simulink model "model"  (R2024b)
settings: Solver=VariableStepAuto  StartTime=0.0  StopTime=inf  RelTol=1e-3
StopFcn:
  | try
  |     delete(instrfindall);
  |     fclose(instrfindall);
  | catch
  | end
libraries: simulink x4, instrumentseriallib x3
settings Model: Creator=andre  LastModifiedBy=andre

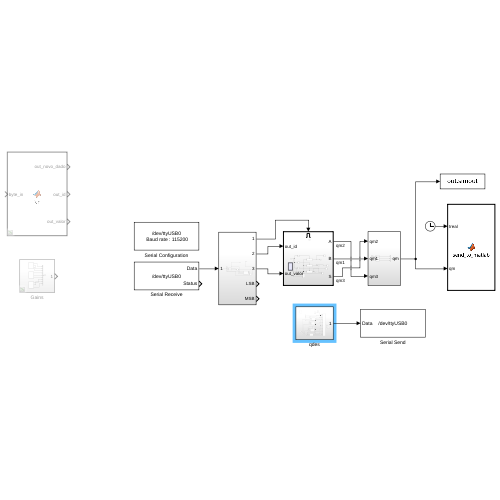
[thumbnail: Simulink's stored preview of the top-level diagram]
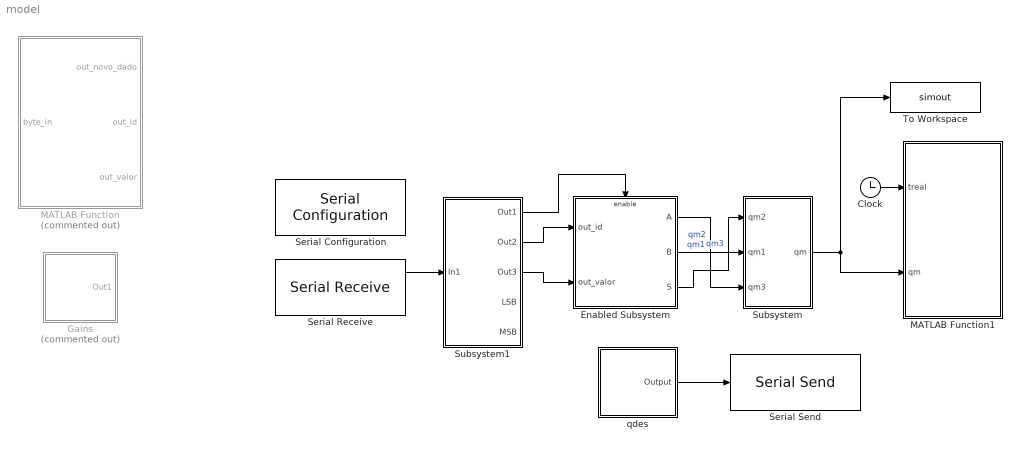
== system model ==
  Clock : Clock
  Enabled Subsystem : Subsystem  TreatAsAtomicUnit=on
  Gains : Subsystem  Commented=on
  MATLAB Function : MATLAB Function  Commented=on  TreatAsAtomicUnit=on
  MATLAB Function1 : MATLAB Function  TreatAsAtomicUnit=on
  Serial Configuration : instrumentseriallib/Serial Configuration  Priority=-200000  PortSel=/dev/ttyUSB0  Port=/dev/ttyUSB0  ComPort=/dev/ttyUSB0  BaudRate=115200  DataBits=8  Parity=none  StopBits=1  ByteOrder=little-endian  FlowControl=none  Timeout=10  SimulateUsing=Interpreted execution  BlockInModel=on  aMode=1
  Serial Receive : instrumentseriallib/Serial Receive  Priority=1  PortSel=/dev/ttyUSB0  Port=/dev/ttyUSB0  ComPort=/dev/ttyUSB0  DataType=uint8  SaveDataType=uint8  ToggleHeader=on  Header=[170]  ToggleDataSize=on  DataSize=[5 1]  ToggleTerminator=on  Terminator=Custom terminator  CustomTerminator=[187]  InputFormat=Column major  EnableBlockingMode=off  ActionDataUnavailable=Output last received value  ActionWhenDataUnavailable=Output last received value  CustomValue=0  SampleTime=0.001  SimulateUsing=Interpreted execution  BlockInModel=on  aMode=1
  Serial Send : instrumentseriallib/Serial Send  Priority=1  PortSel=/dev/ttyUSB0  Port=/dev/ttyUSB0  ComPort=/dev/ttyUSB0  Header=[]  Terminator=<none>  CustomTerminator=[]  EnableBlockingMode=off  SimulateUsing=Interpreted execution  BlockInModel=on  aMode=1
  Subsystem : Subsystem
  Subsystem1 : Subsystem
  To Workspace : ToWorkspace  VariableName=simout  SaveFormat=Timeseries  SampleTime=-1
  qdes : Subsystem
  wires:
  Clock/1 -> MATLAB Function1/1(treal)
  Enabled Subsystem/2(B) -> Subsystem/2(qm1)  "qm1"
  Subsystem/1(qm) -> To Workspace/1, MATLAB Function1/2(qm)
  qdes/1(Output) -> Serial Send/1
  Enabled Subsystem/3(S) -> Subsystem/1(qm2)  "qm3"
  Enabled Subsystem/1(A) -> Subsystem/3(qm3)  "qm2"
  Serial Receive/1 -> Subsystem1/1(In1)
  Subsystem1/1(Out1) -> Enabled Subsystem/Enable
  Subsystem1/2(Out2) -> Enabled Subsystem/1(out_id)
  Subsystem1/3(Out3) -> Enabled Subsystem/2(out_valor)

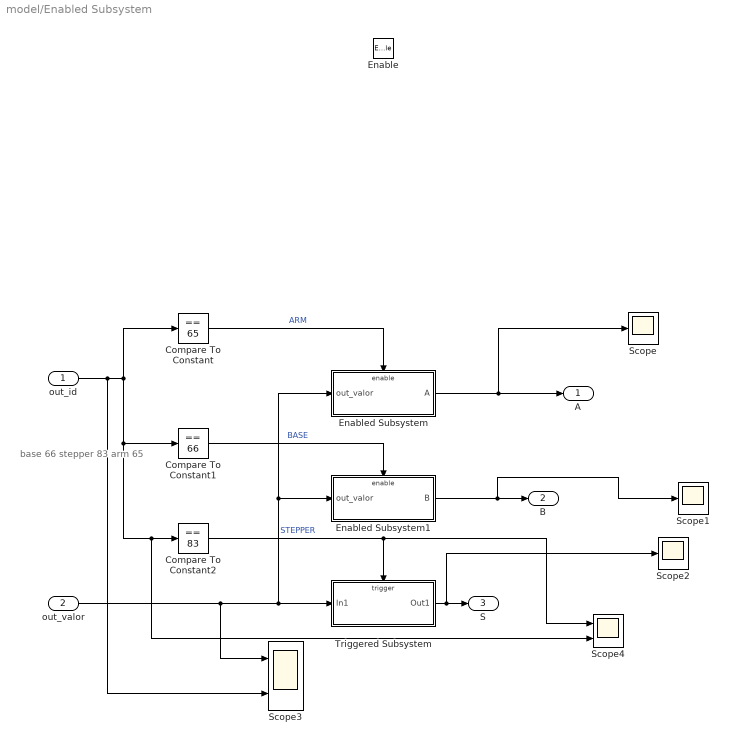
== system model/Enabled Subsystem ==
  note: base 66
      | stepper 83
      | arm 65
  out_id : Inport
  out_valor : Inport  Port=2
  Enable : EnablePort
  Compare To Constant : simulink/Logic and Bit Operations/Compare To Constant  relop===  const=65  OutDataTypeStr=boolean
  Compare To Constant1 : simulink/Logic and Bit Operations/Compare To Constant  relop===  const=66  OutDataTypeStr=boolean
  Compare To Constant2 : simulink/Logic and Bit Operations/Compare To Constant  relop===  const=83  OutDataTypeStr=boolean
  Enabled Subsystem : Subsystem  TreatAsAtomicUnit=on
  Enabled Subsystem1 : Subsystem  TreatAsAtomicUnit=on
  Scope : Scope
  Scope1 : Scope
  Scope2 : Scope
  Scope3 : Scope  NumInputPorts=2
  Scope4 : Scope  NumInputPorts=2
  Triggered Subsystem : Subsystem  TreatAsAtomicUnit=on
  A : Outport
  B : Outport  Port=2
  S : Outport  Port=3
  wires:
  Compare To Constant/1 -> Enabled Subsystem/Enable  "ARM"
  Triggered Subsystem/1(Out1) -> Scope2/1, S/1
  Compare To Constant2/1 -> Scope4/1, Triggered Subsystem/Trigger  "STEPPER"
  out_id/1 -> Scope3/2, Scope4/2, Compare To Constant2/1, Compare To Constant1/1, Compare To Constant/1
  out_valor/1 -> Scope3/1, Triggered Subsystem/1(In1), Enabled Subsystem/1(out_valor), Enabled Subsystem1/1(out_valor)
  Compare To Constant1/1 -> Enabled Subsystem1/Enable  "BASE"
  Enabled Subsystem/1(A) -> Scope/1, A/1
  Enabled Subsystem1/1(B) -> Scope1/1, B/1

== system model/Gains ==
  D_gain : Subsystem
  I_gain : Subsystem
  P_gain : Subsystem
  Vector Concatenate : Concatenate  NumInputs=9
  Out1 : Outport
  wires:
  P_gain/2(Out2) -> Vector Concatenate/2
  P_gain/1(Out1) -> Vector Concatenate/1
  I_gain/2(Out2) -> Vector Concatenate/5
  P_gain/3(Out3) -> Vector Concatenate/3
  I_gain/3(Out3) -> Vector Concatenate/6
  D_gain/1(Out1) -> Vector Concatenate/7
  D_gain/3(Out3) -> Vector Concatenate/9
  D_gain/2(Out2) -> Vector Concatenate/8
  I_gain/1(Out1) -> Vector Concatenate/4
  Vector Concatenate/1 -> Out1/1

== system model/Subsystem ==
  qm2 : Inport
  qm1 : Inport  Port=2
  qm3 : Inport  Port=3
  Cast To Double : DataTypeConversion  OutDataTypeStr=double  SaturateOnIntegerOverflow=off  RndMeth=Floor
  Cast To Double1 : DataTypeConversion  OutDataTypeStr=double  SaturateOnIntegerOverflow=off  RndMeth=Floor
  Cast To Double2 : DataTypeConversion  OutDataTypeStr=double  SaturateOnIntegerOverflow=off  RndMeth=Floor
  Mux : Mux  Inputs=3
  qm : Outport
  wires:
  Mux/1 -> qm/1
  Cast To Double/1 -> Mux/2
  Cast To Double1/1 -> Mux/1
  Cast To Double2/1 -> Mux/3
  qm2/1 -> Cast To Double/1
  qm1/1 -> Cast To Double1/1
  qm3/1 -> Cast To Double2/1

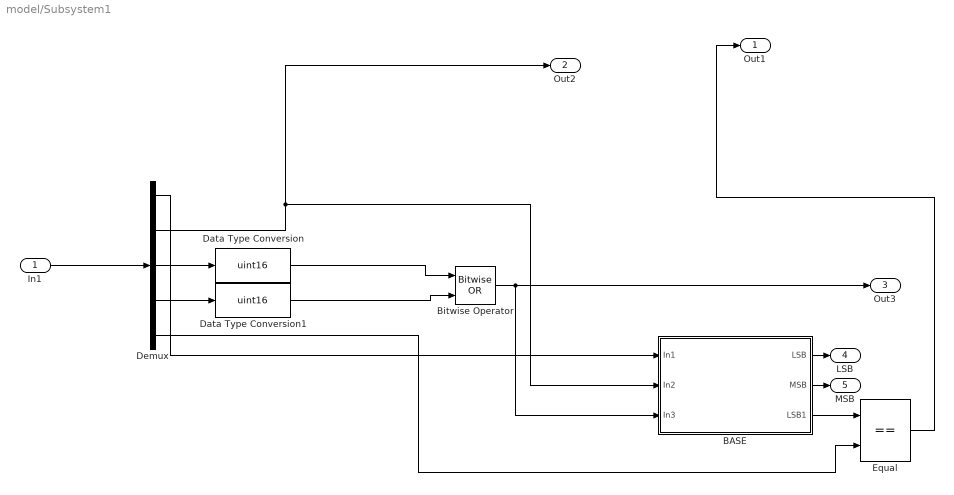
== system model/Subsystem1 ==
  In1 : Inport
  BASE : Subsystem
  Bitwise Operator : simulink/Logic and Bit Operations/Bitwise Operator  logicop=OR  UseBitMask=off  NumInputPorts=2  BitMask=bin2dec('11011001')  BitMaskRealWorld=Stored Integer
  Data Type Conversion : DataTypeConversion  OutDataTypeStr=uint16  SaturateOnIntegerOverflow=off  RndMeth=Floor
  Data Type Conversion1 : DataTypeConversion  OutDataTypeStr=uint16  SaturateOnIntegerOverflow=off  RndMeth=Floor
  Demux : Demux  Outputs=5
  Equal : RelationalOperator  Operator===  OutDataTypeStr=boolean  RndMeth=Simplest  InputSameDT=off
  Out1 : Outport
  Out2 : Outport  Port=2
  Out3 : Outport  Port=3
  LSB : Outport  Port=4
  MSB : Outport  Port=5
  wires:
  Equal/1 -> Out1/1
  Demux/1 -> BASE/1(In1)
  Demux/4 -> Data Type Conversion1/1
  Data Type Conversion/1 -> Bitwise Operator/1
  Data Type Conversion1/1 -> Bitwise Operator/2
  Demux/5 -> Equal/2
  BASE/3(LSB1) -> Equal/1
  Demux/3 -> Data Type Conversion/1
  Bitwise Operator/1 -> Out3/1, BASE/3(In3)
  Demux/2 -> Out2/1, BASE/2(In2)
  BASE/2(MSB) -> MSB/1
  In1/1 -> Demux/1
  BASE/1(LSB) -> LSB/1

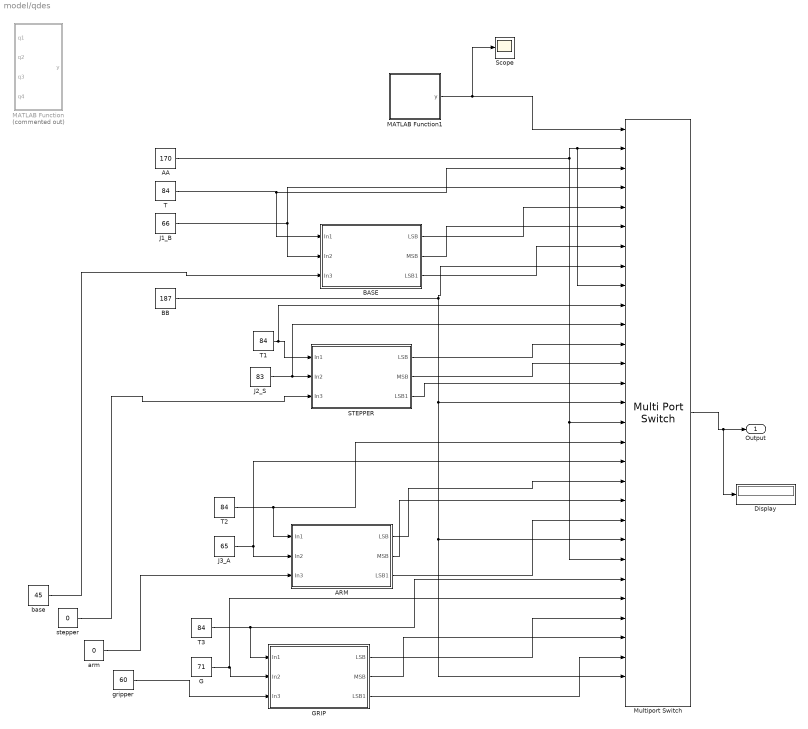
== system model/qdes ==
  AA : Constant  Value=170  OutDataTypeStr=uint8
  ARM : Subsystem
  BASE : Subsystem
  BB : Constant  Value=187  OutDataTypeStr=uint8
  Display : Display
  G : Constant  Value=71  OutDataTypeStr=uint8
  GRIP : Subsystem
  J1_B : Constant  Value=66  OutDataTypeStr=uint8
  J2_S : Constant  Value=83  OutDataTypeStr=uint8
  J3_A : Constant  Value=65  OutDataTypeStr=uint8
  MATLAB Function : MATLAB Function  Commented=on  TreatAsAtomicUnit=on
  MATLAB Function1 : MATLAB Function  TreatAsAtomicUnit=on  SystemSampleTime=.0005
  Multiport Switch : MultiPortSwitch  DataPortOrder=Zero-based contiguous  Inputs=28  DataPortForDefault=Additional data port  zeroidx=on  SaturateOnIntegerOverflow=off  InputSameDT=off
  STEPPER : Subsystem
  Scope : Scope
  T{,1..3} (4 alike) : Constant  Value=84  OutDataTypeStr=uint8
  arm : Constant  Value=0  OutDataTypeStr=uint16
  base : Constant  Value=45  OutDataTypeStr=uint16
  gripper : Constant  Value=60  OutDataTypeStr=uint16
  stepper : Constant  Value=0  OutDataTypeStr=uint16
  Output : Outport
  wires:
  J1_B/1 -> Multiport Switch/4, BASE/2(In2)
  T/1 -> Multiport Switch/3, BASE/1(In1)
  J2_S/1 -> Multiport Switch/11, STEPPER/2(In2)
  J3_A/1 -> Multiport Switch/18, ARM/2(In2)
  T1/1 -> Multiport Switch/10, STEPPER/1(In1)
  T2/1 -> Multiport Switch/17, ARM/1(In1)
  AA/1 -> Multiport Switch/9, Multiport Switch/2, Multiport Switch/23, Multiport Switch/16
  BASE/1(LSB) -> Multiport Switch/5
  BASE/2(MSB) -> Multiport Switch/6
  BASE/3(LSB1) -> Multiport Switch/7
  BB/1 -> Multiport Switch/15, Multiport Switch/29, Multiport Switch/22, Multiport Switch/8
  STEPPER/1(LSB) -> Multiport Switch/12
  STEPPER/2(MSB) -> Multiport Switch/13
  STEPPER/3(LSB1) -> Multiport Switch/14
  ARM/1(LSB) -> Multiport Switch/19
  ARM/2(MSB) -> Multiport Switch/20
  ARM/3(LSB1) -> Multiport Switch/21
  T3/1 -> Multiport Switch/24, GRIP/1(In1)
  G/1 -> Multiport Switch/25, GRIP/2(In2)
  gripper/1 -> GRIP/3(In3)
  GRIP/1(LSB) -> Multiport Switch/26
  GRIP/2(MSB) -> Multiport Switch/27
  GRIP/3(LSB1) -> Multiport Switch/28
  Multiport Switch/1 -> Display/1, Output/1
  arm/1 -> ARM/3(In3)
  stepper/1 -> STEPPER/3(In3)
  base/1 -> BASE/3(In3)
  MATLAB Function1/1(y) -> Scope/1, Multiport Switch/1

== system model/Enabled Subsystem/Enabled Subsystem ==
  out_valor : Inport
  Enable : EnablePort
  A : Outport
  wires:
  out_valor/1 -> A/1

== system model/Enabled Subsystem/Enabled Subsystem1 ==
  out_valor : Inport
  Enable : EnablePort
  B : Outport
  wires:
  out_valor/1 -> B/1

== system model/Enabled Subsystem/Triggered Subsystem ==
  In1 : Inport
  Trigger : TriggerPort  VariantControl=(inherit)
  Out1 : Outport
  wires:
  In1/1 -> Out1/1

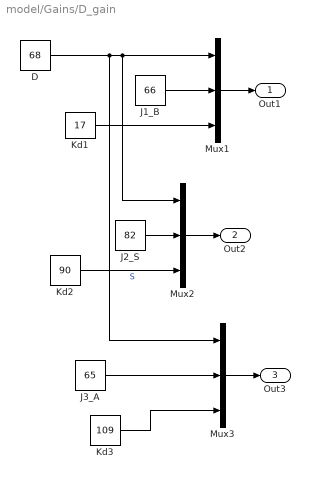
== system model/Gains/D_gain ==
  D : Constant  Value=68  OutDataTypeStr=uint8
  J1_B : Constant  Value=66  OutDataTypeStr=uint8
  J2_S : Constant  Value=82  OutDataTypeStr=uint8
  J3_A : Constant  Value=65  OutDataTypeStr=uint8
  Kd1 : Constant  Value=17  OutDataTypeStr=uint8
  Kd2 : Constant  Value=90  OutDataTypeStr=uint8
  Kd3 : Constant  Value=109  OutDataTypeStr=uint8
  Mux1 : Mux  Inputs=3
  Mux2 : Mux  Inputs=3
  Mux3 : Mux  Inputs=3
  Out1 : Outport
  Out2 : Outport  Port=2
  Out3 : Outport  Port=3
  wires:
  Mux1/1 -> Out1/1
  D/1 -> Mux1/1, Mux2/1, Mux3/1
  Mux3/1 -> Out3/1
  Kd1/1 -> Mux1/3
  J2_S/1 -> Mux2/2
  Mux2/1 -> Out2/1
  J3_A/1 -> Mux3/2
  J1_B/1 -> Mux1/2
  Kd2/1 -> Mux2/3  "S"
  Kd3/1 -> Mux3/3

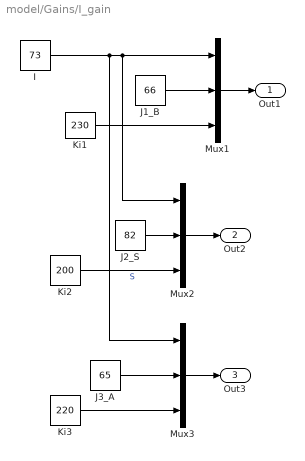
== system model/Gains/I_gain ==
  I : Constant  Value=73  OutDataTypeStr=uint8
  J1_B : Constant  Value=66  OutDataTypeStr=uint8
  J2_S : Constant  Value=82  OutDataTypeStr=uint8
  J3_A : Constant  Value=65  OutDataTypeStr=uint8
  Ki1 : Constant  Value=230  OutDataTypeStr=uint8
  Ki2 : Constant  Value=200  OutDataTypeStr=uint8
  Ki3 : Constant  Value=220  OutDataTypeStr=uint8
  Mux1 : Mux  Inputs=3
  Mux2 : Mux  Inputs=3
  Mux3 : Mux  Inputs=3
  Out1 : Outport
  Out2 : Outport  Port=2
  Out3 : Outport  Port=3
  wires:
  Ki2/1 -> Mux2/3  "S"
  J1_B/1 -> Mux1/2
  J3_A/1 -> Mux3/2
  Mux2/1 -> Out2/1
  J2_S/1 -> Mux2/2
  Mux3/1 -> Out3/1
  Ki3/1 -> Mux3/3
  I/1 -> Mux3/1, Mux2/1, Mux1/1
  Mux1/1 -> Out1/1
  Ki1/1 -> Mux1/3

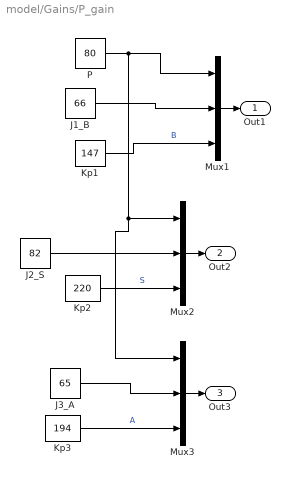
== system model/Gains/P_gain ==
  J1_B : Constant  Value=66  OutDataTypeStr=uint8
  J2_S : Constant  Value=82  OutDataTypeStr=uint8
  J3_A : Constant  Value=65  OutDataTypeStr=uint8
  Kp1 : Constant  Value=147  OutDataTypeStr=uint8
  Kp2 : Constant  Value=220  OutDataTypeStr=uint8
  Kp3 : Constant  Value=194  OutDataTypeStr=uint8
  Mux1 : Mux  Inputs=3
  Mux2 : Mux  Inputs=3
  Mux3 : Mux  Inputs=3
  P : Constant  Value=80  OutDataTypeStr=uint8
  Out1 : Outport
  Out2 : Outport  Port=2
  Out3 : Outport  Port=3
  wires:
  J3_A/1 -> Mux3/2
  J2_S/1 -> Mux2/2
  P/1 -> Mux3/1, Mux2/1, Mux1/1
  Kp1/1 -> Mux1/3  "B"
  Kp2/1 -> Mux2/3  "S"
  J1_B/1 -> Mux1/2
  Mux2/1 -> Out2/1
  Mux1/1 -> Out1/1
  Kp3/1 -> Mux3/3  "A"
  Mux3/1 -> Out3/1

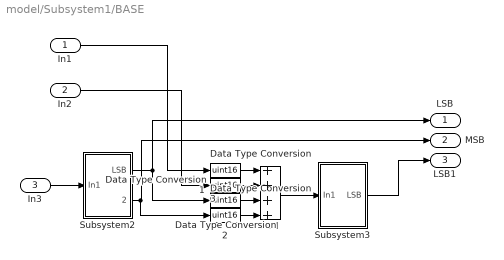
== system model/Subsystem1/BASE ==
  In1 : Inport
  In2 : Inport  Port=2
  In3 : Inport  Port=3
  Add : Sum  Inputs=++++  AccumDataTypeStr=uint16
  Data Type Conversion{,1..3} (4 alike) : DataTypeConversion  OutDataTypeStr=uint16  SaturateOnIntegerOverflow=off  RndMeth=Floor
  Subsystem2 : Subsystem
  Subsystem3 : Subsystem
  LSB : Outport
  MSB : Outport  Port=2
  LSB1 : Outport  Port=3
  wires:
  Add/1 -> Subsystem3/1(In1)
  Subsystem2/1(LSB) -> Data Type Conversion2/1, LSB/1
  Subsystem2/2(MSB) -> Data Type Conversion3/1, MSB/1
  In3/1 -> Subsystem2/1(In1)
  Subsystem3/1(LSB) -> LSB1/1
  Data Type Conversion/1 -> Add/1
  Data Type Conversion1/1 -> Add/2
  Data Type Conversion2/1 -> Add/3
  Data Type Conversion3/1 -> Add/4
  In1/1 -> Data Type Conversion/1
  In2/1 -> Data Type Conversion1/1

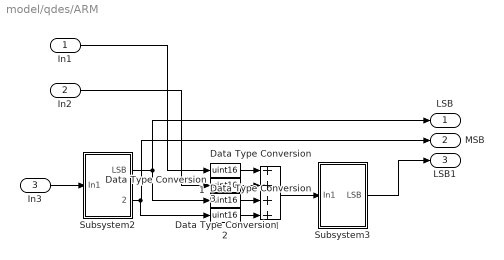
== system model/qdes/ARM ==
  In1 : Inport
  In2 : Inport  Port=2
  In3 : Inport  Port=3
  Add : Sum  Inputs=++++  AccumDataTypeStr=uint16
  Data Type Conversion{,1..3} (4 alike) : DataTypeConversion  OutDataTypeStr=uint16  SaturateOnIntegerOverflow=off  RndMeth=Floor
  Subsystem2 : Subsystem
  Subsystem3 : Subsystem
  LSB : Outport
  MSB : Outport  Port=2
  LSB1 : Outport  Port=3
  wires:
  Add/1 -> Subsystem3/1(In1)
  Subsystem2/1(LSB) -> Data Type Conversion2/1, LSB/1
  Subsystem2/2(MSB) -> Data Type Conversion3/1, MSB/1
  In3/1 -> Subsystem2/1(In1)
  Subsystem3/1(LSB) -> LSB1/1
  Data Type Conversion/1 -> Add/1
  Data Type Conversion1/1 -> Add/2
  Data Type Conversion2/1 -> Add/3
  Data Type Conversion3/1 -> Add/4
  In1/1 -> Data Type Conversion/1
  In2/1 -> Data Type Conversion1/1

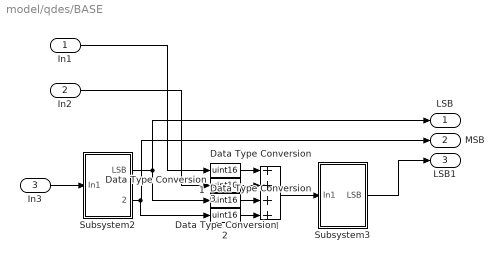
== system model/qdes/BASE ==
  In1 : Inport
  In2 : Inport  Port=2
  In3 : Inport  Port=3
  Add : Sum  Inputs=++++  AccumDataTypeStr=uint16
  Data Type Conversion{,1..3} (4 alike) : DataTypeConversion  OutDataTypeStr=uint16  SaturateOnIntegerOverflow=off  RndMeth=Floor
  Subsystem2 : Subsystem
  Subsystem3 : Subsystem
  LSB : Outport
  MSB : Outport  Port=2
  LSB1 : Outport  Port=3
  wires:
  Add/1 -> Subsystem3/1(In1)
  Subsystem2/1(LSB) -> Data Type Conversion2/1, LSB/1
  Subsystem2/2(MSB) -> Data Type Conversion3/1, MSB/1
  In3/1 -> Subsystem2/1(In1)
  Subsystem3/1(LSB) -> LSB1/1
  Data Type Conversion/1 -> Add/1
  Data Type Conversion1/1 -> Add/2
  Data Type Conversion2/1 -> Add/3
  Data Type Conversion3/1 -> Add/4
  In1/1 -> Data Type Conversion/1
  In2/1 -> Data Type Conversion1/1

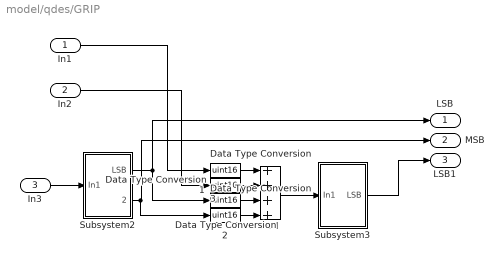
== system model/qdes/GRIP ==
  In1 : Inport
  In2 : Inport  Port=2
  In3 : Inport  Port=3
  Add : Sum  Inputs=++++  AccumDataTypeStr=uint16
  Data Type Conversion{,1..3} (4 alike) : DataTypeConversion  OutDataTypeStr=uint16  SaturateOnIntegerOverflow=off  RndMeth=Floor
  Subsystem2 : Subsystem
  Subsystem3 : Subsystem
  LSB : Outport
  MSB : Outport  Port=2
  LSB1 : Outport  Port=3
  wires:
  Add/1 -> Subsystem3/1(In1)
  Subsystem2/1(LSB) -> Data Type Conversion2/1, LSB/1
  Subsystem2/2(MSB) -> Data Type Conversion3/1, MSB/1
  In3/1 -> Subsystem2/1(In1)
  Subsystem3/1(LSB) -> LSB1/1
  Data Type Conversion/1 -> Add/1
  Data Type Conversion1/1 -> Add/2
  Data Type Conversion2/1 -> Add/3
  Data Type Conversion3/1 -> Add/4
  In1/1 -> Data Type Conversion/1
  In2/1 -> Data Type Conversion1/1

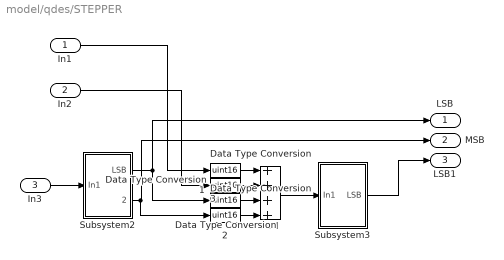
== system model/qdes/STEPPER ==
  In1 : Inport
  In2 : Inport  Port=2
  In3 : Inport  Port=3
  Add : Sum  Inputs=++++  AccumDataTypeStr=uint16
  Data Type Conversion{,1..3} (4 alike) : DataTypeConversion  OutDataTypeStr=uint16  SaturateOnIntegerOverflow=off  RndMeth=Floor
  Subsystem2 : Subsystem
  Subsystem3 : Subsystem
  LSB : Outport
  MSB : Outport  Port=2
  LSB1 : Outport  Port=3
  wires:
  Add/1 -> Subsystem3/1(In1)
  Subsystem2/1(LSB) -> Data Type Conversion2/1, LSB/1
  Subsystem2/2(MSB) -> Data Type Conversion3/1, MSB/1
  In3/1 -> Subsystem2/1(In1)
  Subsystem3/1(LSB) -> LSB1/1
  Data Type Conversion/1 -> Add/1
  Data Type Conversion1/1 -> Add/2
  Data Type Conversion2/1 -> Add/3
  Data Type Conversion3/1 -> Add/4
  In1/1 -> Data Type Conversion/1
  In2/1 -> Data Type Conversion1/1

== system model/Subsystem1/BASE/Subsystem2 ==
  In1 : Inport
  A : DataTypeConversion  OutDataTypeStr=uint8  SaturateOnIntegerOverflow=off  RndMeth=Floor
  Cast To Double : DataTypeConversion  OutDataTypeStr=double  SaturateOnIntegerOverflow=off  RndMeth=Floor
  Constant : Constant  Value=256  OutDataTypeStr=uint16
  Constant1 : Constant  Value=256  OutDataTypeStr=uint16
  Divide : Product  Inputs=*/
  Floor : Rounding
  Math Function : Math  Operator=mod
  S : DataTypeConversion  OutDataTypeStr=uint8  SaturateOnIntegerOverflow=off  RndMeth=Floor
  LSB : Outport
  MSB : Outport  Port=2
  wires:
  Constant1/1 -> Divide/2
  Constant/1 -> Math Function/2
  In1/1 -> Math Function/1, Divide/1
  Floor/1 -> S/1
  Math Function/1 -> A/1
  S/1 -> MSB/1
  A/1 -> LSB/1
  Divide/1 -> Cast To Double/1
  Cast To Double/1 -> Floor/1

== system model/Subsystem1/BASE/Subsystem3 ==
  In1 : Inport
  A : DataTypeConversion  OutDataTypeStr=uint8  SaturateOnIntegerOverflow=off  RndMeth=Floor
  Constant : Constant  Value=256  OutDataTypeStr=uint16
  Math Function : Math  Operator=mod
  LSB : Outport
  wires:
  Constant/1 -> Math Function/2
  In1/1 -> Math Function/1
  Math Function/1 -> A/1
  A/1 -> LSB/1

== system model/qdes/ARM/Subsystem2 ==
  In1 : Inport
  A : DataTypeConversion  OutDataTypeStr=uint8  SaturateOnIntegerOverflow=off  RndMeth=Floor
  Cast To Double : DataTypeConversion  OutDataTypeStr=double  SaturateOnIntegerOverflow=off  RndMeth=Floor
  Constant : Constant  Value=256  OutDataTypeStr=uint16
  Constant1 : Constant  Value=256  OutDataTypeStr=uint16
  Divide : Product  Inputs=*/
  Floor : Rounding
  Math Function : Math  Operator=mod
  S : DataTypeConversion  OutDataTypeStr=uint8  SaturateOnIntegerOverflow=off  RndMeth=Floor
  LSB : Outport
  MSB : Outport  Port=2
  wires:
  Constant1/1 -> Divide/2
  Constant/1 -> Math Function/2
  In1/1 -> Math Function/1, Divide/1
  Floor/1 -> S/1
  Math Function/1 -> A/1
  S/1 -> MSB/1
  A/1 -> LSB/1
  Divide/1 -> Cast To Double/1
  Cast To Double/1 -> Floor/1

== system model/qdes/ARM/Subsystem3 ==
  In1 : Inport
  A : DataTypeConversion  OutDataTypeStr=uint8  SaturateOnIntegerOverflow=off  RndMeth=Floor
  Constant : Constant  Value=256  OutDataTypeStr=uint16
  Math Function : Math  Operator=mod
  LSB : Outport
  wires:
  Constant/1 -> Math Function/2
  In1/1 -> Math Function/1
  Math Function/1 -> A/1
  A/1 -> LSB/1

== system model/qdes/BASE/Subsystem2 ==
  In1 : Inport
  A : DataTypeConversion  OutDataTypeStr=uint8  SaturateOnIntegerOverflow=off  RndMeth=Floor
  Cast To Double : DataTypeConversion  OutDataTypeStr=double  SaturateOnIntegerOverflow=off  RndMeth=Floor
  Constant : Constant  Value=256  OutDataTypeStr=uint16
  Constant1 : Constant  Value=256  OutDataTypeStr=uint16
  Divide : Product  Inputs=*/
  Floor : Rounding
  Math Function : Math  Operator=mod
  S : DataTypeConversion  OutDataTypeStr=uint8  SaturateOnIntegerOverflow=off  RndMeth=Floor
  LSB : Outport
  MSB : Outport  Port=2
  wires:
  Constant1/1 -> Divide/2
  Constant/1 -> Math Function/2
  In1/1 -> Math Function/1, Divide/1
  Floor/1 -> S/1
  Math Function/1 -> A/1
  S/1 -> MSB/1
  A/1 -> LSB/1
  Divide/1 -> Cast To Double/1
  Cast To Double/1 -> Floor/1

== system model/qdes/BASE/Subsystem3 ==
  In1 : Inport
  A : DataTypeConversion  OutDataTypeStr=uint8  SaturateOnIntegerOverflow=off  RndMeth=Floor
  Constant : Constant  Value=256  OutDataTypeStr=uint16
  Math Function : Math  Operator=mod
  LSB : Outport
  wires:
  Constant/1 -> Math Function/2
  In1/1 -> Math Function/1
  Math Function/1 -> A/1
  A/1 -> LSB/1

== system model/qdes/GRIP/Subsystem2 ==
  In1 : Inport
  A : DataTypeConversion  OutDataTypeStr=uint8  SaturateOnIntegerOverflow=off  RndMeth=Floor
  Cast To Double : DataTypeConversion  OutDataTypeStr=double  SaturateOnIntegerOverflow=off  RndMeth=Floor
  Constant : Constant  Value=256  OutDataTypeStr=uint16
  Constant1 : Constant  Value=256  OutDataTypeStr=uint16
  Divide : Product  Inputs=*/
  Floor : Rounding
  Math Function : Math  Operator=mod
  S : DataTypeConversion  OutDataTypeStr=uint8  SaturateOnIntegerOverflow=off  RndMeth=Floor
  LSB : Outport
  MSB : Outport  Port=2
  wires:
  Constant1/1 -> Divide/2
  Constant/1 -> Math Function/2
  In1/1 -> Math Function/1, Divide/1
  Floor/1 -> S/1
  Math Function/1 -> A/1
  S/1 -> MSB/1
  A/1 -> LSB/1
  Divide/1 -> Cast To Double/1
  Cast To Double/1 -> Floor/1

== system model/qdes/GRIP/Subsystem3 ==
  In1 : Inport
  A : DataTypeConversion  OutDataTypeStr=uint8  SaturateOnIntegerOverflow=off  RndMeth=Floor
  Constant : Constant  Value=256  OutDataTypeStr=uint16
  Math Function : Math  Operator=mod
  LSB : Outport
  wires:
  Constant/1 -> Math Function/2
  In1/1 -> Math Function/1
  Math Function/1 -> A/1
  A/1 -> LSB/1

== system model/qdes/STEPPER/Subsystem2 ==
  In1 : Inport
  A : DataTypeConversion  OutDataTypeStr=uint8  SaturateOnIntegerOverflow=off  RndMeth=Floor
  Cast To Double : DataTypeConversion  OutDataTypeStr=double  SaturateOnIntegerOverflow=off  RndMeth=Floor
  Constant : Constant  Value=256  OutDataTypeStr=uint16
  Constant1 : Constant  Value=256  OutDataTypeStr=uint16
  Divide : Product  Inputs=*/
  Floor : Rounding
  Math Function : Math  Operator=mod
  S : DataTypeConversion  OutDataTypeStr=uint8  SaturateOnIntegerOverflow=off  RndMeth=Floor
  LSB : Outport
  MSB : Outport  Port=2
  wires:
  Constant1/1 -> Divide/2
  Constant/1 -> Math Function/2
  In1/1 -> Math Function/1, Divide/1
  Floor/1 -> S/1
  Math Function/1 -> A/1
  S/1 -> MSB/1
  A/1 -> LSB/1
  Divide/1 -> Cast To Double/1
  Cast To Double/1 -> Floor/1

== system model/qdes/STEPPER/Subsystem3 ==
  In1 : Inport
  A : DataTypeConversion  OutDataTypeStr=uint8  SaturateOnIntegerOverflow=off  RndMeth=Floor
  Constant : Constant  Value=256  OutDataTypeStr=uint16
  Math Function : Math  Operator=mod
  LSB : Outport
  wires:
  Constant/1 -> Math Function/2
  In1/1 -> Math Function/1
  Math Function/1 -> A/1
  A/1 -> LSB/1

== matlab function model/MATLAB Function1 ==
  data: treal input; qm input
function send_to_matlab(treal,qm)
    
    assignin('base',"treal",treal);
    assignin('base','qm', qm);

end

== matlab function model/MATLAB Function ==
  data: out_novo_dado output; byte_in input; out_id output; out_valor output
function [out_novo_dado,out_id, out_valor] = fcn(byte_in)
% Esta função implementa a máquina de estados para parsear o frame
% Os 'persistent' são variáveis estáticas (como as 'static' em C)

% --- Definições ---
persistent FRAME_SOF;
persistent FRAME_EOF;
persistent STATE_WAIT_SOF;
persistent STATE_WAIT_CMD;
persistent STATE_WAIT_ID;
persistent STATE_WAIT_VALUE_L;
persistent STATE_WAIT_VALUE_H;
persistent STATE_WAIT_CHK;
persistent STATE_WAIT_EOF;

% --- Variáveis de Estado (estáticas) ---
persistent s_current_state;
persistent s_received_cmd;
persistent s_received_id;
persistent s_received_val_l;
persistent s_received_val_h;

% --- Bloco de Inicialização (só roda 1 vez) ---
if isempty(s_current_state)
    FRAME_SOF = 170; % 0xAA
    FRAME_EOF = 187; % 0xBB
    
    STATE_WAIT_SOF = 0;
    STATE_WAIT_CMD = 1;
    STATE_WAIT_ID = 2;
    STATE_WAIT_VALUE_L = 3;
    STATE_WAIT_VALUE_H = 4;
    STATE_WAIT_CHK = 5;
    STATE_WAIT_EOF = 6;
    
    s_current_state = STATE_WAIT_SOF;
    s_received_cmd = uint8(0);
    s_received_id = uint8(0);
    s_received_val_l = uint8(0);
    s_received_val_h = uint8(0);
end

% Saídas padrão (não temos um frame novo AINDA)
out_id = uint8(0);
out_valor = uint16(0);
out_novo_dado = false; % 'Flag' que diz "dado novo chegou"

% --- A Máquina de Estados ---
switch s_current_state
    case STATE_WAIT_SOF
        if (byte_in == FRAME_SOF)
            s_current_state = STATE_WAIT_CMD;
        end
        
    case STATE_WAIT_CMD
        s_received_cmd = byte_in;
        s_current_state = STATE_WAIT_ID;
        
    case STATE_WAIT_ID
        s_received_id = byte_in;
        s_current_state = STATE_WAIT_VALUE_L;
        
    case STATE_WAIT_VALUE_L
        s_received_val_l = byte_in;
        s_current_state = STATE_WAIT_VALUE_H;

    case STATE_WAIT_VALUE_H
        s_received_val_h = byte_in;
        s_current_state = STATE_WAIT_CHK;
        
    case STATE_WAIT_CHK
        % Recalcula o checksum (igual ao C)
        chk_calc = bitand(uint32(s_received_cmd) + uint32(s_received_id) + uint32(s_received_val_l) + uint32(s_received_val_h), 255);
        
        if (byte_in == chk_calc)
            s_current_state = STATE_WAIT_EOF;
        else
            % Checksum falhou, volte ao início
            s_current_state = STATE_WAIT_SOF;
        end
        
    case STATE_WAIT_EOF
        if (byte_in == FRAME_EOF)
            % FRAME VÁLIDO! Monta as saídas
            out_id = s_received_id;
            
            % Monta o uint16 (Little-Endian)
            out_valor = bitor(bitshift(uint16(s_received_val_h), 8), uint16(s_received_val_l));
            
            % Sinaliza que um novo dado está pronto
            out_novo_dado = true;
        end
        % Se chegou aqui, ou foi sucesso ou falha, volte ao início
        s_current_state = STATE_WAIT_SOF;
end

== matlab function model/qdes/MATLAB Function ==
  data: y output; q1 input; q2 input; q3 input; q4 input
function y = fcn(q1,q2,q3,q4)
% Saída y: índice do MultiportSwitch (0–27)
% Regras:
% - Quando uma junta pede mudança (qk = 1), ela só será ativada
%   DEPOIS que o ciclo atual (0–6) terminar.
% - Prioridade q4 > q3 > q2 > q1.
% - Cada junta transmite índices base..base+6 em loop.

    persistent currentMode counter pendingMode;
    
    % Inicialização
    if isempty(currentMode)
        currentMode = 0;   % nenhuma junta ativa
    end
    if isempty(counter)
        counter = 0;
    end
    if isempty(pendingMode)
        pendingMode = 0;  % pedido aguardando fim do ciclo
    end

    %% ===== 1. CHECAR PEDIDOS DE MUDANÇA =====
    % prioridade: q4 > q3 > q2 > q1
    if q4
        pendingMode = 4;
    elseif q3
        pendingMode = 3;
    elseif q2
        pendingMode = 2;
    elseif q1
        pendingMode = 1;
    end

    %% ===== 2. SE O CICLO ATUAL TERMINOU, APLICAR MUDANÇA =====
    if counter == 0   % só troca quando inicia um novo ciclo 0–6
        if pendingMode ~= 0
            currentMode = pendingMode;
            pendingMode = 0;
        end
    end

    %% ===== 3. DEFINIR BASE DA JUNTA ATUAL =====
    switch currentMode
        case 1
            base = 0;
        case 2
            base = 7;
        case 3
            base = 14;
        case 4
            base = 21;
        otherwise
            base = 0;   % estado inicial
    end

    %% ===== 4. GERAR SAÍDA =====
    y = base + counter;

    %% ===== 5. AVANÇAR CONTADOR (0–6) =====
    counter = counter + 1;
    if counter > 6
        counter = 0;
    end
end

== matlab function model/qdes/MATLAB Function1 ==
  data: y output
function y = fcn

persistent count;
if isempty(count)
    count = 0;
end
y = count;
count = count + 1;
if count == 28
    count = 0;
end

end
